simulink model "PTDHT_2020a"  (R2020a)
settings: Solver=VariableStepAuto  StartTime=0.0  StopTime=10  RelTol=1e-3
settings Model: Creator=Admin  LastModifiedBy=Hp

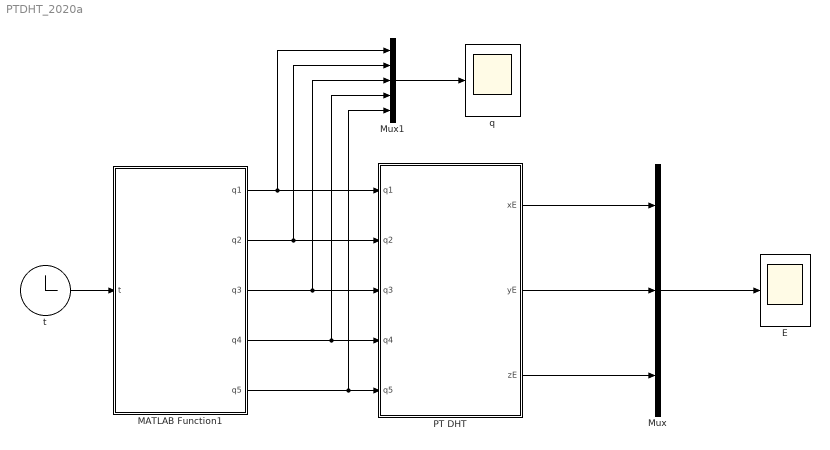
== system PTDHT_2020a ==
  E : Scope
  MATLAB Function1 : MATLAB Function  TreatAsAtomicUnit=on
  Mux : Mux  Inputs=3
  Mux1 : Mux  Inputs=5
  "PT DHT  " : MATLAB Function  TreatAsAtomicUnit=on
  q : Scope
  t : Clock
  wires:
  MATLAB Function1/4(q4) -> "PT DHT  "/4(q4), Mux1/4
  MATLAB Function1/3(q3) -> "PT DHT  "/3(q3), Mux1/3
  MATLAB Function1/2(q2) -> "PT DHT  "/2(q2), Mux1/2
  MATLAB Function1/1(q1) -> "PT DHT  "/1(q1), Mux1/1
  t/1 -> MATLAB Function1/1(t)
  Mux/1 -> E/1
  MATLAB Function1/5(q5) -> Mux1/5, "PT DHT  "/5(q5)
  "PT DHT  "/3(zE) -> Mux/3
  "PT DHT  "/2(yE) -> Mux/2
  "PT DHT  "/1(xE) -> Mux/1
  Mux1/1 -> q/1

== matlab function PTDHT_2020a/MATLAB Function1 ==
  data: t input; q1 output; q2 output; q3 output; q4 output; q5 output
function [q1,q2,q3,q4,q5] = fcn(t)
q1=sin(t)+1;
q2=pi*cos(t);
q3=0.75*(cos(t)+1);
q4=-(pi/6)*cos(t)-(pi/2);
q5=pi*sin(t)
end

== matlab function PTDHT_2020a/PT DHT   ==
  data: q1 input; xE output; q2 input; q3 input; q4 input; yE output; zE output; q5 input
function [xE,yE,zE] = fcn(q1,q2,q3,q4,q5)
%Khai bao thong so 
L1=2;
L2=2;
a2=1;
L3=1.5;
L4=1;
L5=0.75;
%Phuong trinh dong hoc thuan
xE=((L4 + L5) * cos(q4) + a2) * cos(q2) + q1;
yE=sin(q2) * ((L4 + L5) * cos(q4) + a2);
zE=(-L4 - L5) * sin(q4) + q3 + L2;
end
